simulink model "bernuli"  (Simulink 7.9)
settings: Solver=ode45  StartTime=-10.0  StopTime=20.0  RelTol=1e-3
libraries: simulink x1
settings Model: Creator=Mihail  LastModifiedBy=Mihail

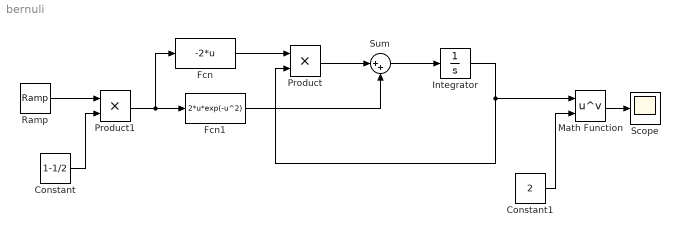
== system bernuli ==
  Constant : Constant  Value=1-1/2
  Constant1 : Constant  Value=2
  Fcn : Fcn  Expr=-2*u
  Fcn1 : Fcn  Expr=2*u*exp(-u^2)
  Integrator : Integrator
  Math Function : Math  Operator=pow  SaturateOnIntegerOverflow=on
  Product : Product  RndMeth=Zero
  Product1 : Product  RndMeth=Zero
  Ramp : simulink/Sources/Ramp  slope=0.1  start=0  X0=1
  Scope : Scope
  Sum : Sum  Inputs=|++
  wires:
  Integrator/1 -> Product/2, Math Function/1
  Product/1 -> Sum/1
  Sum/1 -> Integrator/1
  Fcn/1 -> Product/1
  Fcn1/1 -> Sum/2
  Ramp/1 -> Product1/1
  Product1/1 -> Fcn1/1, Fcn/1
  Constant/1 -> Product1/2
  Constant1/1 -> Math Function/2
  Math Function/1 -> Scope/1
